simulink model "MST_AyrikModel"  (R2022b)
settings: Solver=FixedStepAuto  StartTime=0.0  StopTime=10.0  FixedStep=0.1  RelTol=1e-3
InitFcn:
  | MST_Ayrik
values from neighbouring files (symbols this model uses):
  constants = [fx_now ... (first row only)    [MST_Ayrik.m]    (also in ayrikHesaplar.m)
settings Model: Creator=aysen  LastModifiedBy=aysen

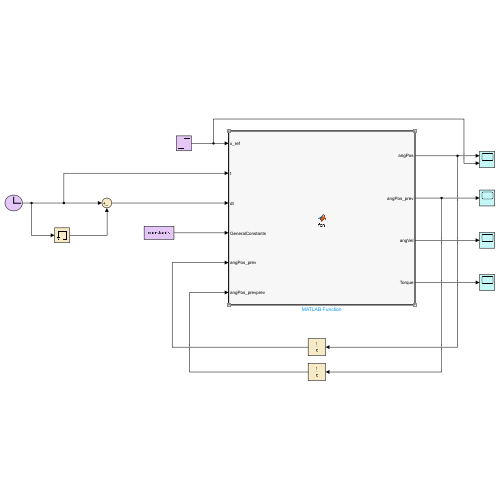
[thumbnail: Simulink's stored preview of the top-level diagram]
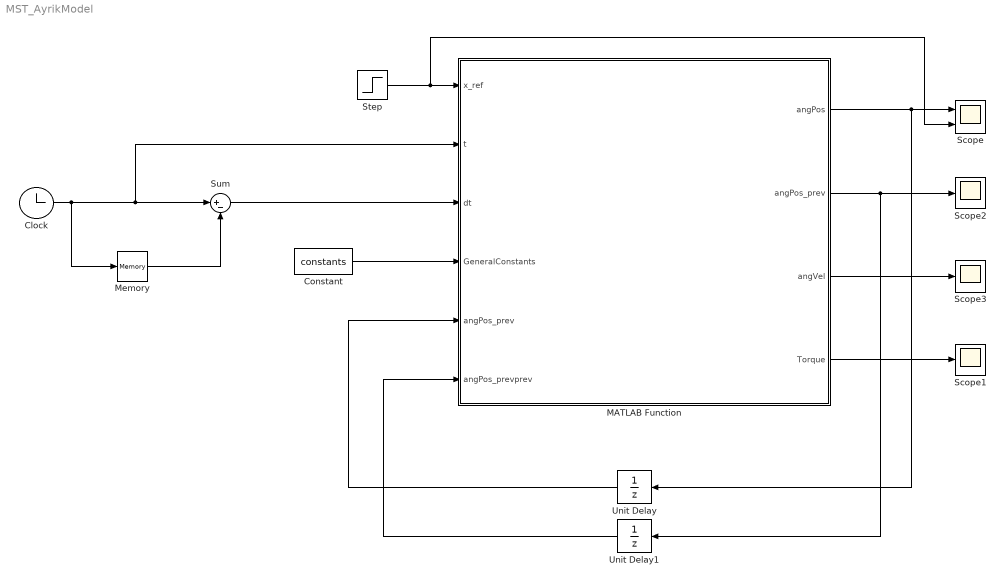
== system MST_AyrikModel ==
  Clock : Clock
  Constant : Constant  Value=constants
  MATLAB Function : MATLAB Function  TreatAsAtomicUnit=on
  Memory : Memory
  Scope : Scope  NumInputPorts=2
  Scope1 : Scope
  Scope2 : Scope
  Scope3 : Scope
  Step : Step  Time=0  After=10  SampleTime=0
  Sum : Sum  Inputs=|+-
  Unit Delay : UnitDelay  SampleTime=-1  HasFrameUpgradeWarning=on
  Unit Delay1 : UnitDelay  SampleTime=-1  HasFrameUpgradeWarning=on
  wires:
  Clock/1 -> Memory/1, MATLAB Function/2(t), Sum/1
  Memory/1 -> Sum/2
  Sum/1 -> MATLAB Function/3(dt)
  Constant/1 -> MATLAB Function/4(GeneralConstants)
  MATLAB Function/1(angPos) -> Scope/1, Unit Delay/1
  MATLAB Function/4(Torque) -> Scope1/1
  Unit Delay/1 -> MATLAB Function/5("angPos_prev ")
  Unit Delay1/1 -> MATLAB Function/6(angPos_prevprev)
  MATLAB Function/2(angPos_prev) -> Unit Delay1/1, Scope2/1
  MATLAB Function/3(angVel) -> Scope3/1
  Step/1 -> Scope/2, MATLAB Function/1(x_ref)

== matlab function MST_AyrikModel/MATLAB Function ==
  data: x_ref input size=1; angPos output size=1; angPos_prev output; angVel output; t input size=1; dt input; GeneralConstants input; Torque output size=1; angPos_prev input size=1; angPos_prevprev input size=1
function [angPos, angPos_prev, angVel, Torque] = fcn(x_ref,t, dt, GeneralConstants, angPos_prev, angPos_prevprev)
fx_now = GeneralConstants(1,1);
fx_pre = GeneralConstants(2,1);
fx_fut = GeneralConstants(3,1);
x_0 = GeneralConstants(4,1);
x_0_dot = GeneralConstants(5, 1);
Ae = GeneralConstants(6, 1);
%N1 = GeneralConstants(7, 1);
%N2 = GeneralConstants(8, 1);
%N3 = GeneralConstants(9, 1);

error = x_ref - angPos_prev;
C1 = x_ref - (((angPos_prev * fx_now) + (angPos_prevprev * fx_pre)) / fx_fut);

if (t == 0)
    angPos = x_0;       
    angVel = 0;
    Torque = 0;

elseif (t == dt)
    Torque = fx_fut * (C1 - (Ae * error));
    angPos = x_0 + x_0_dot * dt;
    angVel = x_0_dot;

else
    Torque = fx_fut * (C1 - (Ae * error));
    angPos = (angPos_prev * fx_now + angPos_prevprev * fx_pre + Torque) / fx_fut;
    angVel = (angPos - angPos_prevprev) / (2 * dt);
    Torque = Torque * 1000;
end
